simulink model "HybridControllerD3D3"  (Simulink 7.5)
settings: Solver=FixedStepDiscrete  StartTime=0.0  StopTime=inf  FixedStep=samplePeriod  RelTol=1e-3  AbsTol=1e-6
PreLoadFcn:
  | initializeSimulation;
InitFcn:
  | clear('all');
  | initializeSimulation;
values from neighbouring files (symbols this model uses):
  damperA = 0    [initializeSimulation.m]
  damperB = 0    [initializeSimulation.m]
  damperC = 0    [initializeSimulation.m]
  damperCanon = 1    [initializeSimulation.m]
  flowCanon = 3.85    [initializeSimulation.m]
  forceCanon = 1    [initializeSimulation.m]
  frictionA = 0    [initializeSimulation.m]
  frictionB = 0    [initializeSimulation.m]
  frictionC = 0    [initializeSimulation.m]
  gasConstant = 1.8    [initializeSimulation.m]
  lengthCanon = 1    [initializeSimulation.m]
  massA = 4.2    [initializeSimulation.m]
  massB = 2.5    [initializeSimulation.m]
  massC = 2.5    [initializeSimulation.m]
  massCanon = 0.002588    [initializeSimulation.m]
  maxDisplA = (stroke2A + endLength2A) * lengthCanon    (= 22)    [initializeSimulation.m]
  maxDisplB = (stroke2B + endLength2B) * lengthCanon    (= 42)    [initializeSimulation.m]
  maxDisplC = (stroke2C + endLength2C) * lengthCanon    (= 72)    [initializeSimulation.m]
  maxOilVolume = volume * (1 - (precharge/supplyPress)^(1/gasConstant))    (= 10.5071802963)    [initializeSimulation.m]
  maxVelocA = (maxFlowA * flowCanon / (area1A * areaCanon)) / velocCanon    [initializeSimulation.m]
  maxVelocB = (maxFlowB * flowCanon / (area1B * areaCanon)) / velocCanon    [initializeSimulation.m]
  maxVelocC = (maxFlowC * flowCanon / (area1C * areaCanon)) / velocCanon    [initializeSimulation.m]
  minDisplA = -(stroke1A + endLength1A) * lengthCanon    (= -22)    [initializeSimulation.m]
  minDisplB = -(stroke1B + endLength1B) * lengthCanon    (= -42)    [initializeSimulation.m]
  minDisplC = -(stroke1C + endLength1C) * lengthCanon    (= -72)    [initializeSimulation.m]
  minVelocA = -(maxFlowA * flowCanon / (area2A * areaCanon)) / velocCanon    [initializeSimulation.m]
  minVelocB = -(maxFlowB * flowCanon / (area2B * areaCanon)) / velocCanon    [initializeSimulation.m]
  minVelocC = -(maxFlowC * flowCanon / (area2C * areaCanon)) / velocCanon    [initializeSimulation.m]
  nAct = 8    [initializeSimulation.m]
  nAdcU = 12    [initializeSimulation.m]
  nDinp = 4    [initializeSimulation.m]
  nDout = 4    [initializeSimulation.m]
  nDucU = 8    [initializeSimulation.m]
  nEncU = 2    [initializeSimulation.m]
  precharge = 1000    [initializeSimulation.m]
  pumpFlow = 1e10    (= 10000000000)    [initializeSimulation.m]
  returnPress = 50    [initializeSimulation.m]
  staticForceA = 0    [initializeSimulation.m]
  staticForceB = 0    [initializeSimulation.m]
  staticForceC = 0    [initializeSimulation.m]
  supplyPress = 3000    [initializeSimulation.m]
  velocCanon = 1    [initializeSimulation.m]
  volume = accumVolume * accumNumber    (= 23)    [initializeSimulation.m]
  volumeCanon = 231    [initializeSimulation.m]
  yieldDisplA = 0.1    [initializeSimulation.m]
  yieldDisplB = 0.1    [initializeSimulation.m]
  yieldDisplC = 0.1    [initializeSimulation.m]
undefined symbols (not defined in the file or in its folder): DiscIntNeverNeededParam, HybridCtrlParameters
libraries: simulink x2
(part 3 of 3)

== system HybridControllerD3D3/model/ActuatorPayloadMdl/static channel #3/payload/friction ==
  veloc : Inport  OutDataType=sfix(16)  OutScaling=2^0
  1-beta : Gain  Gain=1-hysteresis  ParameterDataType=sfix(16)  ParameterScaling=2^0  OutDataType=sfix(16)  OutScaling=2^0  SaturateOnIntegerOverflow=on  OutDataTypeStr=Inherit: Same as input  ParamDataTypeStr=Inherit: Same as input
  Sign : Signum
  Sum : Sum  Inputs=|++  OutDataType=sfix(16)  OutScaling=2^0  SaturateOnIntegerOverflow=on
  Sum1 : Sum  Inputs=|+-  OutDataType=sfix(16)  OutScaling=2^0  SaturateOnIntegerOverflow=on
  beta : Constant  Value=hysteresis  OutDataType=sfix(16)  OutScaling=2^0
  integrator : DiscreteIntegrator  SampleTime=-1  OutDataType=sfix(16)  OutScaling=2^0  LimitOutput=on  UpperSaturationLimit=1  LowerSaturationLimit=-1  ICPrevOutput=DiscIntNeverNeededParam  ICPrevScaledInput=DiscIntNeverNeededParam
  one : Constant  OutDataType=sfix(16)  OutScaling=2^0
  prod1 : Product  OutDataType=sfix(16)  OutScaling=2^0  SaturateOnIntegerOverflow=on  InputSameDT=on  OutDataTypeStr=Inherit: Same as first input
  prod2 : Product  OutDataType=sfix(16)  OutScaling=2^0  SaturateOnIntegerOverflow=on  InputSameDT=on  OutDataTypeStr=Inherit: Same as first input
  prod3 : Product  Inputs=3  OutDataType=sfix(16)  OutScaling=2^0  SaturateOnIntegerOverflow=on  InputSameDT=on  OutDataTypeStr=Inherit: Same as first input
  prod4 : Product  OutDataType=sfix(16)  OutScaling=2^0  SaturateOnIntegerOverflow=on  InputSameDT=on  OutDataTypeStr=Inherit: Same as first input
  sliding friction : Constant  Value=friction  OutDataType=sfix(16)  OutScaling=2^0
  y inv : Gain  Gain=1/max(eps, yieldDispl)  ParameterDataType=sfix(16)  ParameterScaling=2^0  OutDataType=sfix(16)  OutScaling=2^0  SaturateOnIntegerOverflow=on  OutDataTypeStr=Inherit: Same as input  ParamDataTypeStr=Inherit: Same as input
  force : Outport  OutDataType=sfix(16)  OutScaling=2^0
  wires:
  sliding friction/1 -> prod1/1
  prod1/1 -> force/1
  veloc/1 -> prod4/2, prod2/2
  prod4/1 -> Sign/1
  Sign/1 -> 1-beta/1
  1-beta/1 -> Sum/2
  beta/1 -> Sum/1
  Sum/1 -> prod3/3
  one/1 -> Sum1/1
  prod3/1 -> Sum1/2
  Sum1/1 -> prod2/1
  prod2/1 -> y inv/1
  y inv/1 -> integrator/1
  integrator/1 -> prod1/2, prod4/1, prod3/1, prod3/2  "zee"

== system HybridControllerD3D3/model/ActuatorPayloadMdl/static channel #4/payload/double integrator ==
  accel : Inport
  displ gen : DiscreteIntegrator  IntegratorMethod=Integration: Backward Euler  SampleTime=-1  OutDataType=sfix(16)  OutScaling=2^0  LimitOutput=on  UpperSaturationLimit=maxDisplC  LowerSaturationLimit=minDisplC  ShowSaturationPort=on  ICPrevOutput=DiscIntNeverNeededParam  ICPrevScaledInput=DiscIntNeverNeededParam
  veloc gen : Subsystem  mask{maxVeloc=maxVelocC*velocCanon, minVeloc=minVelocC*velocCanon, maxDispl=maxDisplC, minDispl=minDisplC}
      mask prompts: maxVeloc "Max velocity"; minVeloc "Min velocity"; maxDispl "Max displacement"; minDispl "Min displacement"
  displ : Outport
  veloc : Outport  Port=2
  acc : Outport  Port=3
  wires:
  displ gen/2 -> veloc gen/3(reset)
  displ gen/1 -> displ/1, veloc gen/2(displ)
  veloc gen/1(veloc) -> displ gen/1, veloc/1
  accel/1 -> veloc gen/1(accel), acc/1

== system HybridControllerD3D3/model/ActuatorPayloadMdl/static channel #4/payload/friction ==
  veloc : Inport  OutDataType=sfix(16)  OutScaling=2^0
  1-beta : Gain  Gain=1-hysteresis  ParameterDataType=sfix(16)  ParameterScaling=2^0  OutDataType=sfix(16)  OutScaling=2^0  SaturateOnIntegerOverflow=on  OutDataTypeStr=Inherit: Same as input  ParamDataTypeStr=Inherit: Same as input
  Sign : Signum
  Sum : Sum  Inputs=|++  OutDataType=sfix(16)  OutScaling=2^0  SaturateOnIntegerOverflow=on
  Sum1 : Sum  Inputs=|+-  OutDataType=sfix(16)  OutScaling=2^0  SaturateOnIntegerOverflow=on
  beta : Constant  Value=hysteresis  OutDataType=sfix(16)  OutScaling=2^0
  integrator : DiscreteIntegrator  SampleTime=-1  OutDataType=sfix(16)  OutScaling=2^0  LimitOutput=on  UpperSaturationLimit=1  LowerSaturationLimit=-1  ICPrevOutput=DiscIntNeverNeededParam  ICPrevScaledInput=DiscIntNeverNeededParam
  one : Constant  OutDataType=sfix(16)  OutScaling=2^0
  prod1 : Product  OutDataType=sfix(16)  OutScaling=2^0  SaturateOnIntegerOverflow=on  InputSameDT=on  OutDataTypeStr=Inherit: Same as first input
  prod2 : Product  OutDataType=sfix(16)  OutScaling=2^0  SaturateOnIntegerOverflow=on  InputSameDT=on  OutDataTypeStr=Inherit: Same as first input
  prod3 : Product  Inputs=3  OutDataType=sfix(16)  OutScaling=2^0  SaturateOnIntegerOverflow=on  InputSameDT=on  OutDataTypeStr=Inherit: Same as first input
  prod4 : Product  OutDataType=sfix(16)  OutScaling=2^0  SaturateOnIntegerOverflow=on  InputSameDT=on  OutDataTypeStr=Inherit: Same as first input
  sliding friction : Constant  Value=friction  OutDataType=sfix(16)  OutScaling=2^0
  y inv : Gain  Gain=1/max(eps, yieldDispl)  ParameterDataType=sfix(16)  ParameterScaling=2^0  OutDataType=sfix(16)  OutScaling=2^0  SaturateOnIntegerOverflow=on  OutDataTypeStr=Inherit: Same as input  ParamDataTypeStr=Inherit: Same as input
  force : Outport  OutDataType=sfix(16)  OutScaling=2^0
  wires:
  sliding friction/1 -> prod1/1
  prod1/1 -> force/1
  veloc/1 -> prod4/2, prod2/2
  prod4/1 -> Sign/1
  Sign/1 -> 1-beta/1
  1-beta/1 -> Sum/2
  beta/1 -> Sum/1
  Sum/1 -> prod3/3
  one/1 -> Sum1/1
  prod3/1 -> Sum1/2
  Sum1/1 -> prod2/1
  prod2/1 -> y inv/1
  y inv/1 -> integrator/1
  integrator/1 -> prod1/2, prod4/1, prod3/1, prod3/2  "zee"

== system HybridControllerD3D3/model/simPC HC/SubSystem1/Subsystem/If Action Subsystem1 ==
  In1 : Inport  OutDataType=fixdt(1, 16)  OutScaling=2^0
  In2 : Inport  Port=2  OutDataType=fixdt(1, 16)  OutScaling=2^0
  Action Port : ActionPort  ActionType=then
  Relational Operator : RelationalOperator  Operator===  LogicOutDataTypeMode=boolean  LogicDataType=fixdt(0, 8)  OutDataTypeStr=boolean
  Out1 : Outport  OutDataType=fixdt(1, 16)  OutScaling=2^0
  wires:
  Relational Operator/1 -> Out1/1
  In1/1 -> Relational Operator/1
  In2/1 -> Relational Operator/2

== system HybridControllerD3D3/model/simPC HC/SubSystem1/Subsystem/If Action Subsystem2 ==
  In1 : Inport  OutDataType=fixdt(1, 16)  OutScaling=2^0
  In2 : Inport  Port=2  OutDataType=fixdt(1, 16)  OutScaling=2^0
  Action Port : ActionPort  ActionType=else
  Relational Operator : RelationalOperator  Operator===  LogicOutDataTypeMode=boolean  LogicDataType=fixdt(0, 8)  OutDataTypeStr=boolean
  Out1 : Outport  OutDataType=fixdt(1, 16)  OutScaling=2^0
  wires:
  Relational Operator/1 -> Out1/1
  In1/1 -> Relational Operator/1
  In2/1 -> Relational Operator/2

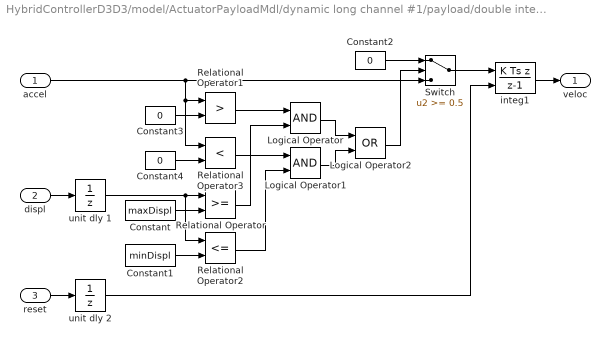
== system HybridControllerD3D3/model/ActuatorPayloadMdl/dynamic long channel #1/payload/double integrator/veloc gen ==
  accel : Inport  OutDataType=sfix(16)  OutScaling=2^0
  displ : Inport  Port=2  OutDataType=sfix(16)  OutScaling=2^0
  reset : Inport  Port=3  OutDataType=sfix(16)  OutScaling=2^0
  Constant : Constant  Value=maxDispl  OutDataType=sfix(16)  OutScaling=2^0
  Constant1 : Constant  Value=minDispl  OutDataType=sfix(16)  OutScaling=2^0
  Constant2 : Constant  Value=0  OutDataType=sfix(16)  OutScaling=2^0
  Constant3 : Constant  Value=0  OutDataType=sfix(16)  OutScaling=2^0
  Constant4 : Constant  Value=0  OutDataType=sfix(16)  OutScaling=2^0
  Logical Operator : Logic
  Logical Operator1 : Logic
  Logical Operator2 : Logic  Operator=OR
  Relational Operator : RelationalOperator  InputSameDT=on
  Relational Operator1 : RelationalOperator  Operator=>  InputSameDT=on
  Relational Operator2 : RelationalOperator  Operator=<=  InputSameDT=on
  Relational Operator3 : RelationalOperator  Operator=<  InputSameDT=on
  Switch : Switch  Threshold=0.5  SaturateOnIntegerOverflow=on  InputSameDT=on
  integ1 : DiscreteIntegrator  IntegratorMethod=Integration: Backward Euler  ExternalReset=either  SampleTime=-1  OutDataType=sfix(16)  OutScaling=2^0  LimitOutput=on  UpperSaturationLimit=maxVeloc  LowerSaturationLimit=minVeloc  ICPrevOutput=DiscIntNeverNeededParam  ICPrevScaledInput=DiscIntNeverNeededParam
  unit dly 1 : UnitDelay  SampleTime=-1
  unit dly 2 : UnitDelay  SampleTime=-1
  veloc : Outport  OutDataType=sfix(16)  OutScaling=2^0
  wires:
  unit dly 1/1 -> Relational Operator2/1, Relational Operator/1
  reset/1 -> unit dly 2/1
  displ/1 -> unit dly 1/1
  Logical Operator1/1 -> Logical Operator2/2
  unit dly 2/1 -> integ1/2
  Switch/1 -> integ1/1
  Logical Operator2/1 -> Switch/2
  Constant2/1 -> Switch/1
  Logical Operator/1 -> Logical Operator2/1
  Relational Operator3/1 -> Logical Operator1/1
  Constant4/1 -> Relational Operator3/2
  Relational Operator1/1 -> Logical Operator/1
  Constant3/1 -> Relational Operator1/2
  accel/1 -> Switch/3, Relational Operator1/1, Relational Operator3/1
  Constant1/1 -> Relational Operator2/2
  Relational Operator2/1 -> Logical Operator1/2
  Relational Operator/1 -> Logical Operator/2
  Constant/1 -> Relational Operator/2
  integ1/1 -> veloc/1

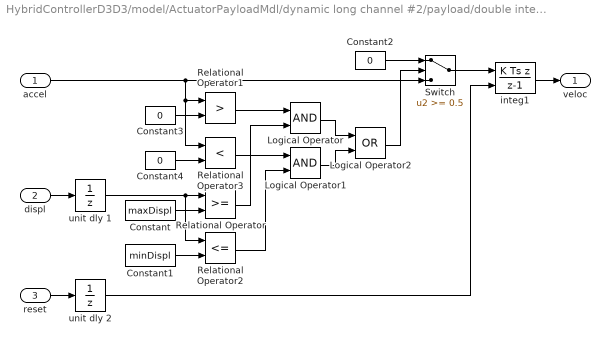
== system HybridControllerD3D3/model/ActuatorPayloadMdl/dynamic long channel #2/payload/double integrator/veloc gen ==
  accel : Inport  OutDataType=sfix(16)  OutScaling=2^0
  displ : Inport  Port=2  OutDataType=sfix(16)  OutScaling=2^0
  reset : Inport  Port=3  OutDataType=sfix(16)  OutScaling=2^0
  Constant : Constant  Value=maxDispl  OutDataType=sfix(16)  OutScaling=2^0
  Constant1 : Constant  Value=minDispl  OutDataType=sfix(16)  OutScaling=2^0
  Constant2 : Constant  Value=0  OutDataType=sfix(16)  OutScaling=2^0
  Constant3 : Constant  Value=0  OutDataType=sfix(16)  OutScaling=2^0
  Constant4 : Constant  Value=0  OutDataType=sfix(16)  OutScaling=2^0
  Logical Operator : Logic
  Logical Operator1 : Logic
  Logical Operator2 : Logic  Operator=OR
  Relational Operator : RelationalOperator  InputSameDT=on
  Relational Operator1 : RelationalOperator  Operator=>  InputSameDT=on
  Relational Operator2 : RelationalOperator  Operator=<=  InputSameDT=on
  Relational Operator3 : RelationalOperator  Operator=<  InputSameDT=on
  Switch : Switch  Threshold=0.5  SaturateOnIntegerOverflow=on  InputSameDT=on
  integ1 : DiscreteIntegrator  IntegratorMethod=Integration: Backward Euler  ExternalReset=either  SampleTime=-1  OutDataType=sfix(16)  OutScaling=2^0  LimitOutput=on  UpperSaturationLimit=maxVeloc  LowerSaturationLimit=minVeloc  ICPrevOutput=DiscIntNeverNeededParam  ICPrevScaledInput=DiscIntNeverNeededParam
  unit dly 1 : UnitDelay  SampleTime=-1
  unit dly 2 : UnitDelay  SampleTime=-1
  veloc : Outport  OutDataType=sfix(16)  OutScaling=2^0
  wires:
  unit dly 1/1 -> Relational Operator2/1, Relational Operator/1
  reset/1 -> unit dly 2/1
  displ/1 -> unit dly 1/1
  Logical Operator1/1 -> Logical Operator2/2
  unit dly 2/1 -> integ1/2
  Switch/1 -> integ1/1
  Logical Operator2/1 -> Switch/2
  Constant2/1 -> Switch/1
  Logical Operator/1 -> Logical Operator2/1
  Relational Operator3/1 -> Logical Operator1/1
  Constant4/1 -> Relational Operator3/2
  Relational Operator1/1 -> Logical Operator/1
  Constant3/1 -> Relational Operator1/2
  accel/1 -> Switch/3, Relational Operator1/1, Relational Operator3/1
  Constant1/1 -> Relational Operator2/2
  Relational Operator2/1 -> Logical Operator1/2
  Relational Operator/1 -> Logical Operator/2
  Constant/1 -> Relational Operator/2
  integ1/1 -> veloc/1

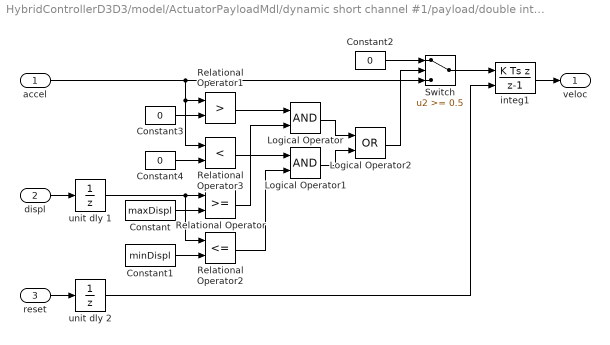
== system HybridControllerD3D3/model/ActuatorPayloadMdl/dynamic short channel #1/payload/double integrator/veloc gen ==
  accel : Inport  OutDataType=sfix(16)  OutScaling=2^0
  displ : Inport  Port=2  OutDataType=sfix(16)  OutScaling=2^0
  reset : Inport  Port=3  OutDataType=sfix(16)  OutScaling=2^0
  Constant : Constant  Value=maxDispl  OutDataType=sfix(16)  OutScaling=2^0
  Constant1 : Constant  Value=minDispl  OutDataType=sfix(16)  OutScaling=2^0
  Constant2 : Constant  Value=0  OutDataType=sfix(16)  OutScaling=2^0
  Constant3 : Constant  Value=0  OutDataType=sfix(16)  OutScaling=2^0
  Constant4 : Constant  Value=0  OutDataType=sfix(16)  OutScaling=2^0
  Logical Operator : Logic
  Logical Operator1 : Logic
  Logical Operator2 : Logic  Operator=OR
  Relational Operator : RelationalOperator  InputSameDT=on
  Relational Operator1 : RelationalOperator  Operator=>  InputSameDT=on
  Relational Operator2 : RelationalOperator  Operator=<=  InputSameDT=on
  Relational Operator3 : RelationalOperator  Operator=<  InputSameDT=on
  Switch : Switch  Threshold=0.5  SaturateOnIntegerOverflow=on  InputSameDT=on
  integ1 : DiscreteIntegrator  IntegratorMethod=Integration: Backward Euler  ExternalReset=either  SampleTime=-1  OutDataType=sfix(16)  OutScaling=2^0  LimitOutput=on  UpperSaturationLimit=maxVeloc  LowerSaturationLimit=minVeloc  ICPrevOutput=DiscIntNeverNeededParam  ICPrevScaledInput=DiscIntNeverNeededParam
  unit dly 1 : UnitDelay  SampleTime=-1
  unit dly 2 : UnitDelay  SampleTime=-1
  veloc : Outport  OutDataType=sfix(16)  OutScaling=2^0
  wires:
  unit dly 1/1 -> Relational Operator2/1, Relational Operator/1
  reset/1 -> unit dly 2/1
  displ/1 -> unit dly 1/1
  Logical Operator1/1 -> Logical Operator2/2
  unit dly 2/1 -> integ1/2
  Switch/1 -> integ1/1
  Logical Operator2/1 -> Switch/2
  Constant2/1 -> Switch/1
  Logical Operator/1 -> Logical Operator2/1
  Relational Operator3/1 -> Logical Operator1/1
  Constant4/1 -> Relational Operator3/2
  Relational Operator1/1 -> Logical Operator/1
  Constant3/1 -> Relational Operator1/2
  accel/1 -> Switch/3, Relational Operator1/1, Relational Operator3/1
  Constant1/1 -> Relational Operator2/2
  Relational Operator2/1 -> Logical Operator1/2
  Relational Operator/1 -> Logical Operator/2
  Constant/1 -> Relational Operator/2
  integ1/1 -> veloc/1

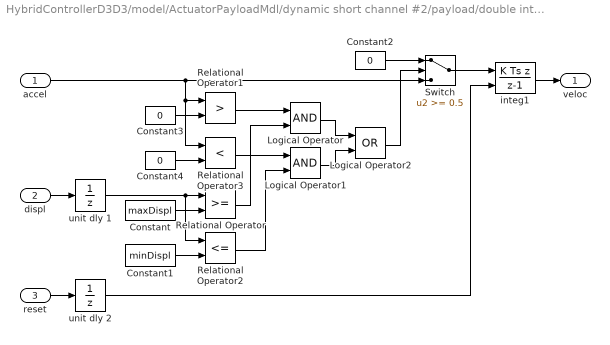
== system HybridControllerD3D3/model/ActuatorPayloadMdl/dynamic short channel #2/payload/double integrator/veloc gen ==
  accel : Inport  OutDataType=sfix(16)  OutScaling=2^0
  displ : Inport  Port=2  OutDataType=sfix(16)  OutScaling=2^0
  reset : Inport  Port=3  OutDataType=sfix(16)  OutScaling=2^0
  Constant : Constant  Value=maxDispl  OutDataType=sfix(16)  OutScaling=2^0
  Constant1 : Constant  Value=minDispl  OutDataType=sfix(16)  OutScaling=2^0
  Constant2 : Constant  Value=0  OutDataType=sfix(16)  OutScaling=2^0
  Constant3 : Constant  Value=0  OutDataType=sfix(16)  OutScaling=2^0
  Constant4 : Constant  Value=0  OutDataType=sfix(16)  OutScaling=2^0
  Logical Operator : Logic
  Logical Operator1 : Logic
  Logical Operator2 : Logic  Operator=OR
  Relational Operator : RelationalOperator  InputSameDT=on
  Relational Operator1 : RelationalOperator  Operator=>  InputSameDT=on
  Relational Operator2 : RelationalOperator  Operator=<=  InputSameDT=on
  Relational Operator3 : RelationalOperator  Operator=<  InputSameDT=on
  Switch : Switch  Threshold=0.5  SaturateOnIntegerOverflow=on  InputSameDT=on
  integ1 : DiscreteIntegrator  IntegratorMethod=Integration: Backward Euler  ExternalReset=either  SampleTime=-1  OutDataType=sfix(16)  OutScaling=2^0  LimitOutput=on  UpperSaturationLimit=maxVeloc  LowerSaturationLimit=minVeloc  ICPrevOutput=DiscIntNeverNeededParam  ICPrevScaledInput=DiscIntNeverNeededParam
  unit dly 1 : UnitDelay  SampleTime=-1
  unit dly 2 : UnitDelay  SampleTime=-1
  veloc : Outport  OutDataType=sfix(16)  OutScaling=2^0
  wires:
  unit dly 1/1 -> Relational Operator2/1, Relational Operator/1
  reset/1 -> unit dly 2/1
  displ/1 -> unit dly 1/1
  Logical Operator1/1 -> Logical Operator2/2
  unit dly 2/1 -> integ1/2
  Switch/1 -> integ1/1
  Logical Operator2/1 -> Switch/2
  Constant2/1 -> Switch/1
  Logical Operator/1 -> Logical Operator2/1
  Relational Operator3/1 -> Logical Operator1/1
  Constant4/1 -> Relational Operator3/2
  Relational Operator1/1 -> Logical Operator/1
  Constant3/1 -> Relational Operator1/2
  accel/1 -> Switch/3, Relational Operator1/1, Relational Operator3/1
  Constant1/1 -> Relational Operator2/2
  Relational Operator2/1 -> Logical Operator1/2
  Relational Operator/1 -> Logical Operator/2
  Constant/1 -> Relational Operator/2
  integ1/1 -> veloc/1

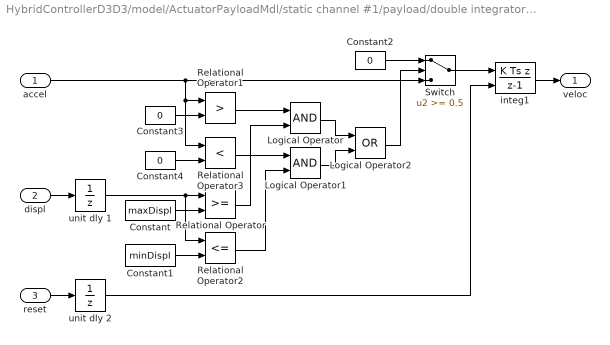
== system HybridControllerD3D3/model/ActuatorPayloadMdl/static channel #1/payload/double integrator/veloc gen ==
  accel : Inport  OutDataType=sfix(16)  OutScaling=2^0
  displ : Inport  Port=2  OutDataType=sfix(16)  OutScaling=2^0
  reset : Inport  Port=3  OutDataType=sfix(16)  OutScaling=2^0
  Constant : Constant  Value=maxDispl  OutDataType=sfix(16)  OutScaling=2^0
  Constant1 : Constant  Value=minDispl  OutDataType=sfix(16)  OutScaling=2^0
  Constant2 : Constant  Value=0  OutDataType=sfix(16)  OutScaling=2^0
  Constant3 : Constant  Value=0  OutDataType=sfix(16)  OutScaling=2^0
  Constant4 : Constant  Value=0  OutDataType=sfix(16)  OutScaling=2^0
  Logical Operator : Logic
  Logical Operator1 : Logic
  Logical Operator2 : Logic  Operator=OR
  Relational Operator : RelationalOperator  InputSameDT=on
  Relational Operator1 : RelationalOperator  Operator=>  InputSameDT=on
  Relational Operator2 : RelationalOperator  Operator=<=  InputSameDT=on
  Relational Operator3 : RelationalOperator  Operator=<  InputSameDT=on
  Switch : Switch  Threshold=0.5  SaturateOnIntegerOverflow=on  InputSameDT=on
  integ1 : DiscreteIntegrator  IntegratorMethod=Integration: Backward Euler  ExternalReset=either  SampleTime=-1  OutDataType=sfix(16)  OutScaling=2^0  LimitOutput=on  UpperSaturationLimit=maxVeloc  LowerSaturationLimit=minVeloc  ICPrevOutput=DiscIntNeverNeededParam  ICPrevScaledInput=DiscIntNeverNeededParam
  unit dly 1 : UnitDelay  SampleTime=-1
  unit dly 2 : UnitDelay  SampleTime=-1
  veloc : Outport  OutDataType=sfix(16)  OutScaling=2^0
  wires:
  unit dly 1/1 -> Relational Operator2/1, Relational Operator/1
  reset/1 -> unit dly 2/1
  displ/1 -> unit dly 1/1
  Logical Operator1/1 -> Logical Operator2/2
  unit dly 2/1 -> integ1/2
  Switch/1 -> integ1/1
  Logical Operator2/1 -> Switch/2
  Constant2/1 -> Switch/1
  Logical Operator/1 -> Logical Operator2/1
  Relational Operator3/1 -> Logical Operator1/1
  Constant4/1 -> Relational Operator3/2
  Relational Operator1/1 -> Logical Operator/1
  Constant3/1 -> Relational Operator1/2
  accel/1 -> Switch/3, Relational Operator1/1, Relational Operator3/1
  Constant1/1 -> Relational Operator2/2
  Relational Operator2/1 -> Logical Operator1/2
  Relational Operator/1 -> Logical Operator/2
  Constant/1 -> Relational Operator/2
  integ1/1 -> veloc/1

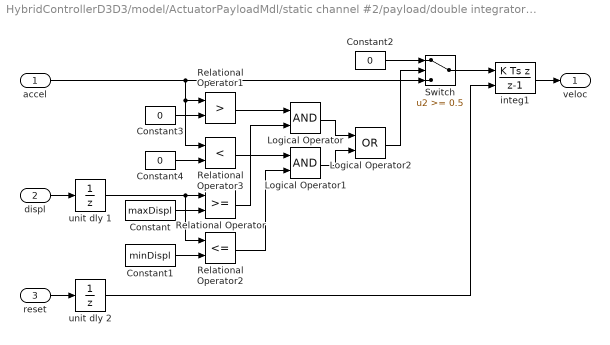
== system HybridControllerD3D3/model/ActuatorPayloadMdl/static channel #2/payload/double integrator/veloc gen ==
  accel : Inport  OutDataType=sfix(16)  OutScaling=2^0
  displ : Inport  Port=2  OutDataType=sfix(16)  OutScaling=2^0
  reset : Inport  Port=3  OutDataType=sfix(16)  OutScaling=2^0
  Constant : Constant  Value=maxDispl  OutDataType=sfix(16)  OutScaling=2^0
  Constant1 : Constant  Value=minDispl  OutDataType=sfix(16)  OutScaling=2^0
  Constant2 : Constant  Value=0  OutDataType=sfix(16)  OutScaling=2^0
  Constant3 : Constant  Value=0  OutDataType=sfix(16)  OutScaling=2^0
  Constant4 : Constant  Value=0  OutDataType=sfix(16)  OutScaling=2^0
  Logical Operator : Logic
  Logical Operator1 : Logic
  Logical Operator2 : Logic  Operator=OR
  Relational Operator : RelationalOperator  InputSameDT=on
  Relational Operator1 : RelationalOperator  Operator=>  InputSameDT=on
  Relational Operator2 : RelationalOperator  Operator=<=  InputSameDT=on
  Relational Operator3 : RelationalOperator  Operator=<  InputSameDT=on
  Switch : Switch  Threshold=0.5  SaturateOnIntegerOverflow=on  InputSameDT=on
  integ1 : DiscreteIntegrator  IntegratorMethod=Integration: Backward Euler  ExternalReset=either  SampleTime=-1  OutDataType=sfix(16)  OutScaling=2^0  LimitOutput=on  UpperSaturationLimit=maxVeloc  LowerSaturationLimit=minVeloc  ICPrevOutput=DiscIntNeverNeededParam  ICPrevScaledInput=DiscIntNeverNeededParam
  unit dly 1 : UnitDelay  SampleTime=-1
  unit dly 2 : UnitDelay  SampleTime=-1
  veloc : Outport  OutDataType=sfix(16)  OutScaling=2^0
  wires:
  unit dly 1/1 -> Relational Operator2/1, Relational Operator/1
  reset/1 -> unit dly 2/1
  displ/1 -> unit dly 1/1
  Logical Operator1/1 -> Logical Operator2/2
  unit dly 2/1 -> integ1/2
  Switch/1 -> integ1/1
  Logical Operator2/1 -> Switch/2
  Constant2/1 -> Switch/1
  Logical Operator/1 -> Logical Operator2/1
  Relational Operator3/1 -> Logical Operator1/1
  Constant4/1 -> Relational Operator3/2
  Relational Operator1/1 -> Logical Operator/1
  Constant3/1 -> Relational Operator1/2
  accel/1 -> Switch/3, Relational Operator1/1, Relational Operator3/1
  Constant1/1 -> Relational Operator2/2
  Relational Operator2/1 -> Logical Operator1/2
  Relational Operator/1 -> Logical Operator/2
  Constant/1 -> Relational Operator/2
  integ1/1 -> veloc/1

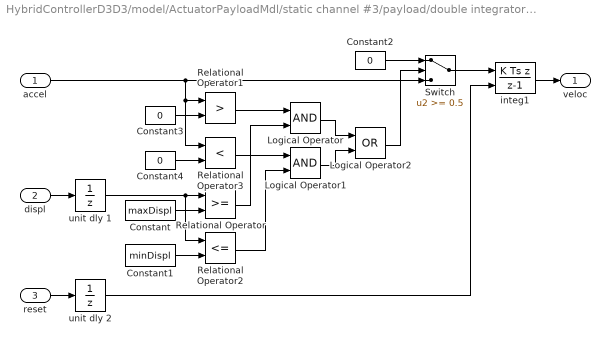
== system HybridControllerD3D3/model/ActuatorPayloadMdl/static channel #3/payload/double integrator/veloc gen ==
  accel : Inport  OutDataType=sfix(16)  OutScaling=2^0
  displ : Inport  Port=2  OutDataType=sfix(16)  OutScaling=2^0
  reset : Inport  Port=3  OutDataType=sfix(16)  OutScaling=2^0
  Constant : Constant  Value=maxDispl  OutDataType=sfix(16)  OutScaling=2^0
  Constant1 : Constant  Value=minDispl  OutDataType=sfix(16)  OutScaling=2^0
  Constant2 : Constant  Value=0  OutDataType=sfix(16)  OutScaling=2^0
  Constant3 : Constant  Value=0  OutDataType=sfix(16)  OutScaling=2^0
  Constant4 : Constant  Value=0  OutDataType=sfix(16)  OutScaling=2^0
  Logical Operator : Logic
  Logical Operator1 : Logic
  Logical Operator2 : Logic  Operator=OR
  Relational Operator : RelationalOperator  InputSameDT=on
  Relational Operator1 : RelationalOperator  Operator=>  InputSameDT=on
  Relational Operator2 : RelationalOperator  Operator=<=  InputSameDT=on
  Relational Operator3 : RelationalOperator  Operator=<  InputSameDT=on
  Switch : Switch  Threshold=0.5  SaturateOnIntegerOverflow=on  InputSameDT=on
  integ1 : DiscreteIntegrator  IntegratorMethod=Integration: Backward Euler  ExternalReset=either  SampleTime=-1  OutDataType=sfix(16)  OutScaling=2^0  LimitOutput=on  UpperSaturationLimit=maxVeloc  LowerSaturationLimit=minVeloc  ICPrevOutput=DiscIntNeverNeededParam  ICPrevScaledInput=DiscIntNeverNeededParam
  unit dly 1 : UnitDelay  SampleTime=-1
  unit dly 2 : UnitDelay  SampleTime=-1
  veloc : Outport  OutDataType=sfix(16)  OutScaling=2^0
  wires:
  unit dly 1/1 -> Relational Operator2/1, Relational Operator/1
  reset/1 -> unit dly 2/1
  displ/1 -> unit dly 1/1
  Logical Operator1/1 -> Logical Operator2/2
  unit dly 2/1 -> integ1/2
  Switch/1 -> integ1/1
  Logical Operator2/1 -> Switch/2
  Constant2/1 -> Switch/1
  Logical Operator/1 -> Logical Operator2/1
  Relational Operator3/1 -> Logical Operator1/1
  Constant4/1 -> Relational Operator3/2
  Relational Operator1/1 -> Logical Operator/1
  Constant3/1 -> Relational Operator1/2
  accel/1 -> Switch/3, Relational Operator1/1, Relational Operator3/1
  Constant1/1 -> Relational Operator2/2
  Relational Operator2/1 -> Logical Operator1/2
  Relational Operator/1 -> Logical Operator/2
  Constant/1 -> Relational Operator/2
  integ1/1 -> veloc/1

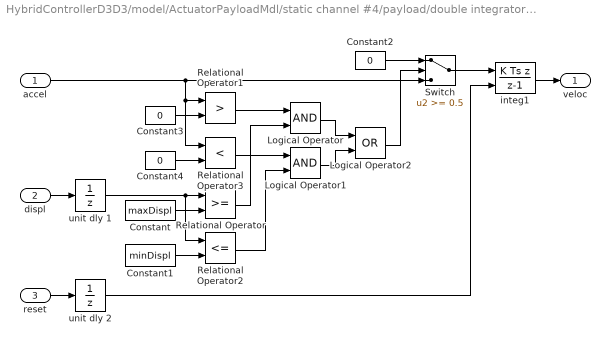
== system HybridControllerD3D3/model/ActuatorPayloadMdl/static channel #4/payload/double integrator/veloc gen ==
  accel : Inport  OutDataType=sfix(16)  OutScaling=2^0
  displ : Inport  Port=2  OutDataType=sfix(16)  OutScaling=2^0
  reset : Inport  Port=3  OutDataType=sfix(16)  OutScaling=2^0
  Constant : Constant  Value=maxDispl  OutDataType=sfix(16)  OutScaling=2^0
  Constant1 : Constant  Value=minDispl  OutDataType=sfix(16)  OutScaling=2^0
  Constant2 : Constant  Value=0  OutDataType=sfix(16)  OutScaling=2^0
  Constant3 : Constant  Value=0  OutDataType=sfix(16)  OutScaling=2^0
  Constant4 : Constant  Value=0  OutDataType=sfix(16)  OutScaling=2^0
  Logical Operator : Logic
  Logical Operator1 : Logic
  Logical Operator2 : Logic  Operator=OR
  Relational Operator : RelationalOperator  InputSameDT=on
  Relational Operator1 : RelationalOperator  Operator=>  InputSameDT=on
  Relational Operator2 : RelationalOperator  Operator=<=  InputSameDT=on
  Relational Operator3 : RelationalOperator  Operator=<  InputSameDT=on
  Switch : Switch  Threshold=0.5  SaturateOnIntegerOverflow=on  InputSameDT=on
  integ1 : DiscreteIntegrator  IntegratorMethod=Integration: Backward Euler  ExternalReset=either  SampleTime=-1  OutDataType=sfix(16)  OutScaling=2^0  LimitOutput=on  UpperSaturationLimit=maxVeloc  LowerSaturationLimit=minVeloc  ICPrevOutput=DiscIntNeverNeededParam  ICPrevScaledInput=DiscIntNeverNeededParam
  unit dly 1 : UnitDelay  SampleTime=-1
  unit dly 2 : UnitDelay  SampleTime=-1
  veloc : Outport  OutDataType=sfix(16)  OutScaling=2^0
  wires:
  unit dly 1/1 -> Relational Operator2/1, Relational Operator/1
  reset/1 -> unit dly 2/1
  displ/1 -> unit dly 1/1
  Logical Operator1/1 -> Logical Operator2/2
  unit dly 2/1 -> integ1/2
  Switch/1 -> integ1/1
  Logical Operator2/1 -> Switch/2
  Constant2/1 -> Switch/1
  Logical Operator/1 -> Logical Operator2/1
  Relational Operator3/1 -> Logical Operator1/1
  Constant4/1 -> Relational Operator3/2
  Relational Operator1/1 -> Logical Operator/1
  Constant3/1 -> Relational Operator1/2
  accel/1 -> Switch/3, Relational Operator1/1, Relational Operator3/1
  Constant1/1 -> Relational Operator2/2
  Relational Operator2/1 -> Logical Operator1/2
  Relational Operator/1 -> Logical Operator/2
  Constant/1 -> Relational Operator/2
  integ1/1 -> veloc/1

== stateflow chart model/simPC HC/Predictor-Corrector ==
  state HybridController [parallel]
    settings: executionOrder=1
    state Predict
      en: state = 1;
      en: setCurDsp(com,i/N);
      en: diSD = 1;
      en: i = 1; iSD = 0;
      en: predictD3(com,i/N);
      du: i++;
      du: predictD3(com,i/N);
    state Initialize
      en: i = 1; iSD = 0;
      en: diSD = 1;
      en: initData(nAct,dtCon);
      en: zeroDsp(com);
    state AutoSlowDown
      en: state = 2;
      en: diSD = 4-i/(0.2*N);
      en: i += diSD; iSD = i;
      en: predictD3(com,i/N);
      du: diSD = 4-i/(0.2*N);
      du: i += diSD; iSD = i;
      du: predictD3(com,i/N);
    state Correct
      en: state = 0;
      en: setCurDsp(com,i/N);
      en: dspLocal = dsp; setNewDsp(dspLocal);
      en: di = min(max(diSD+1/(0.2*N)*(i-iSD),0.001),1.0);
      en: i = min(i+di,N);
      en: correctD3(com,i/N);
      du: di = min(max(diSD+1/(0.2*N)*(i-iSD),0.001),1.0);
      du: i = min(i+di,N);
      du: correctD3(com,i/N);
    Correct -> Predict : [i>=N]
    (default) -> Initialize
    Predict -> Correct [order 2] : [flag==1]
    Initialize -> Correct : [flag==1]
    AutoSlowDown -> Correct : [flag==1]
    Predict -> AutoSlowDown [order 1] : [i>=0.6*N && flag~=1]
  data: dsp input double size=nAct+1; flag input double size=1; com output double size=nAct+1; state output double size=1; i output double size=1; N local double size=1; nAct parameter double size=1 =1; di local double size=1; diSD local double size=1; iSD local double size=1; dspLocal local double size=nAct+1
